simulink model "TermProject_sim"  (R2022a)
settings: Solver=VariableStepAuto  StartTime=0.0  StopTime=3  RelTol=1e-3
values from neighbouring files (symbols this model uses):
  Beq = Jeq/t    (= 0.00458272318505)    [TermProject.m]
  degtorad = pi/180    (= 0.0174532925199)    [TermProject.m]
  Jeq = J+k*JG+k*J_load    (= 1.72310391758e-05)    [TermProject.m]
  Ka_c = 1/Kp_c    (= 1.20938406605)    [TermProject.m]
  Ka_s = 1/Kp_s    (= 31.5427366344)    [TermProject.m]
  Kd_p = wcp/wcs    (= 0.1)    [TermProject.m]
  Ke = Kt    (= 0.0683)    [TermProject.m]
  Ki_c = wcc*Ra    (= 2211.68122813)    [TermProject.m]
  Ki_s = Beq*wcs/Kt    (= 8.43165416785)    [TermProject.m]
  Kp_c = wcc*La    (= 0.826867186425)    [TermProject.m]
  Kp_p = wcp    (= 12.5663706144)    [TermProject.m]
  Kp_s = Jeq*wcs/Kt    (= 0.0317030196711)    [TermProject.m]
  Kt = 68.3*(10^-3)    (= 0.0683)    [TermProject.m]
  La = 0.000658    [TermProject.m]
  N1 = 1    [TermProject.m]
  N2 = 81    [TermProject.m]
  Ra = 1.76    [TermProject.m]
  radtodeg = 180/pi    (= 57.2957795131)    [TermProject.m]
settings Model: Creator=OS  LastModifiedBy=OS

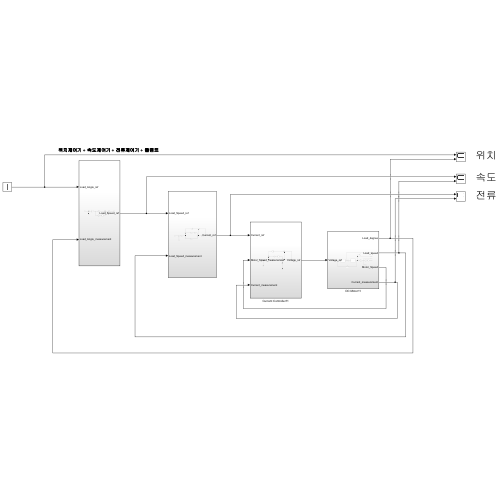
[thumbnail: Simulink's stored preview of the top-level diagram]
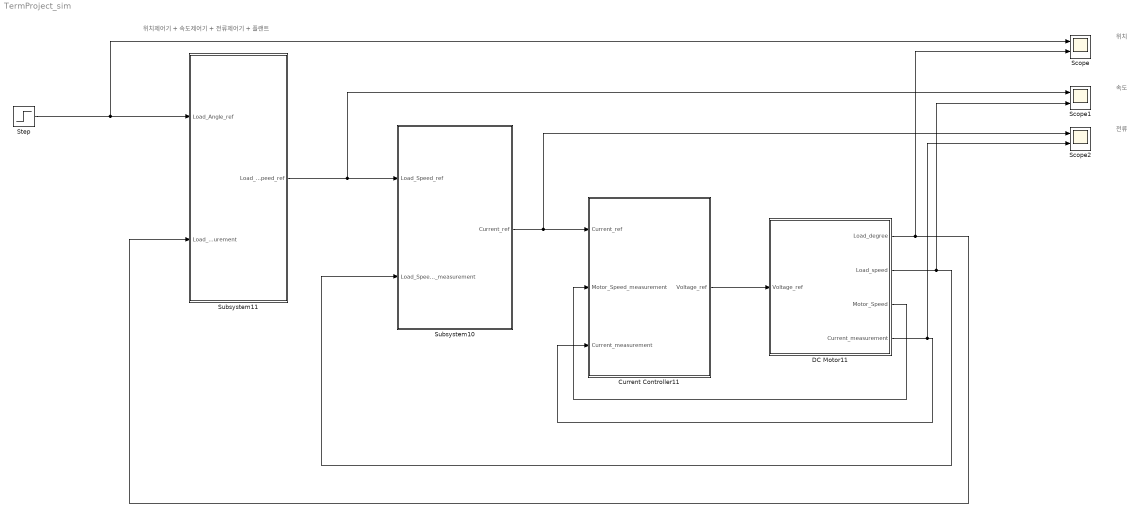
== system TermProject_sim ==
  note: 위치
  note: 위치제어기 + 속도제어기 + 전류제어기 + 플랜트
  note: 속도
  note: 전류
  Current Controller11 : Subsystem
  DC Motor11 : Subsystem
  Scope : Scope  NumInputPorts=2
  Scope1 : Scope  NumInputPorts=2
  Scope2 : Scope  NumInputPorts=2
  Step : Step  After=90  SampleTime=0
  Subsystem10 : Subsystem
  Subsystem11 : Subsystem
  wires:
  DC Motor11/3(Motor_Speed) -> Current Controller11/2(Motor_Speed_measurement)
  Current Controller11/1(Voltage_ref) -> DC Motor11/1(Voltage_ref)
  DC Motor11/4(Current_measurement) -> Scope2/2, Current Controller11/3(Current_measurement)
  DC Motor11/2(Load_speed) -> Scope1/2, Subsystem10/2(Load_Speed_measurement)
  DC Motor11/1(Load_degree) -> Scope/2, Subsystem11/2(Load_Angle_measurement)
  Step/1 -> Subsystem11/1(Load_Angle_ref), Scope/1
  Subsystem10/1(Current_ref) -> Scope2/1, Current Controller11/1(Current_ref)
  Subsystem11/1(Load_Speed_ref) -> Scope1/1, Subsystem10/1(Load_Speed_ref)

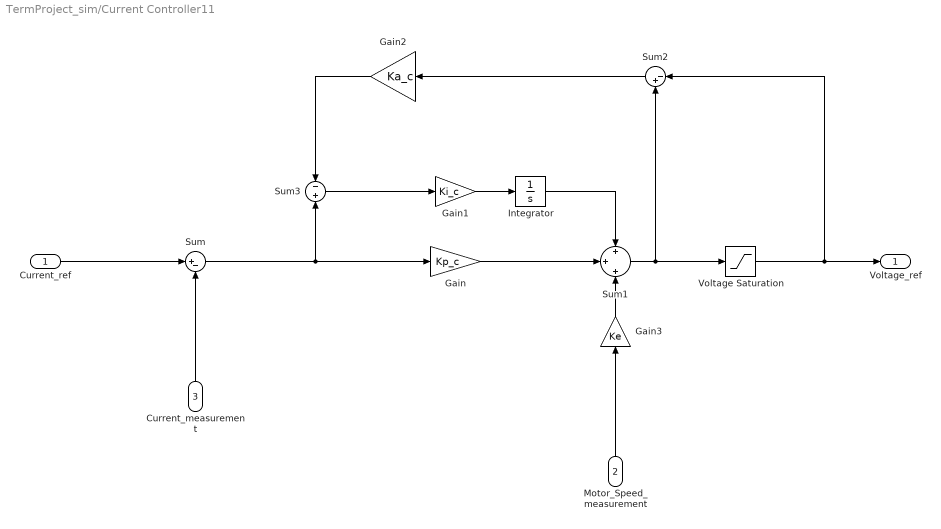
== system TermProject_sim/Current Controller11 ==
  Current_ref : Inport
  Motor_Speed_measurement : Inport  Port=2
  Current_measurement : Inport  Port=3
  Gain : Gain  Gain=Kp_c
  Gain1 : Gain  Gain=Ki_c
  Gain2 : Gain  Gain=Ka_c
  Gain3 : Gain  Gain=Ke
  Integrator : Integrator
  Sum : Sum  Inputs=|+-
  Sum1 : Sum  Inputs=+|+|+
  Sum2 : Sum  Inputs=|-+
  Sum3 : Sum  Inputs=-|+
  Voltage Saturation : Saturate  UpperLimit=48  LowerLimit=-48
  Voltage_ref : Outport
  wires:
  Current_measurement/1 -> Sum/2
  Motor_Speed_measurement/1 -> Gain3/1
  Gain3/1 -> Sum1/3
  Sum2/1 -> Gain2/1
  Gain2/1 -> Sum3/1
  Sum3/1 -> Gain1/1
  Voltage Saturation/1 -> Voltage_ref/1, Sum2/1
  Sum1/1 -> Voltage Saturation/1, Sum2/2
  Gain/1 -> Sum1/2
  Integrator/1 -> Sum1/1
  Gain1/1 -> Integrator/1
  Sum/1 -> Sum3/2, Gain/1
  Current_ref/1 -> Sum/1

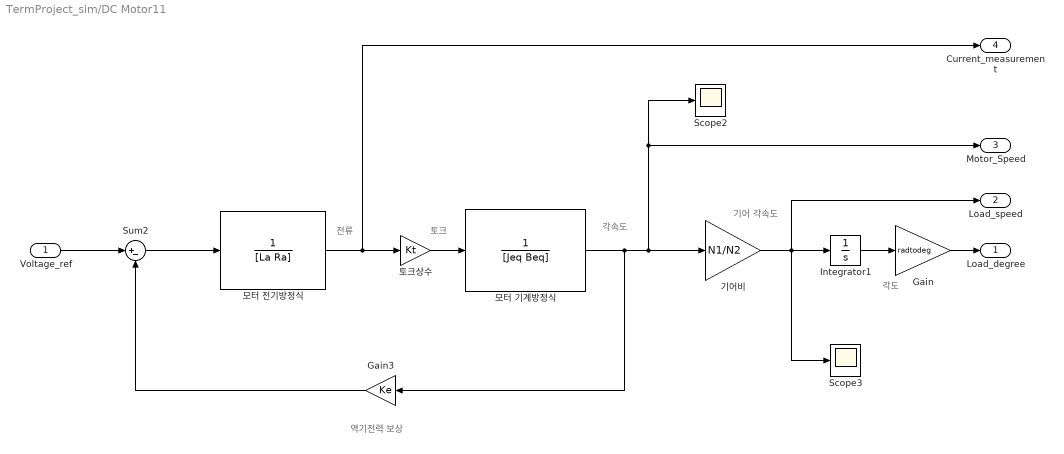
== system TermProject_sim/DC Motor11 ==
  note: 기어 각속도
  note: 각속도
  note: 전류
  note: 토크
  note: 역기전력 보상
  note: 각도
  Voltage_ref : Inport
  Gain : Gain  Gain=radtodeg
  Gain3 : Gain  Gain=Ke
  Integrator1 : Integrator
  Scope2 : Scope
  Scope3 : Scope
  Sum2 : Sum  Inputs=|+-
  기어비 : Gain  Gain=N1/N2
  모터 기계방정식 : TransferFcn  Denominator=[Jeq Beq]
  모터 전기방정식 : TransferFcn  Denominator=[La Ra]
  토크상수 : Gain  Gain=Kt
  Load_degree : Outport
  Load_speed : Outport  Port=2
  Motor_Speed : Outport  Port=3
  Current_measurement : Outport  Port=4
  wires:
  Gain/1 -> Load_degree/1
  Integrator1/1 -> Gain/1
  모터 기계방정식/1 -> Gain3/1, 기어비/1, Motor_Speed/1, Scope2/1
  토크상수/1 -> 모터 기계방정식/1
  Sum2/1 -> 모터 전기방정식/1
  기어비/1 -> Integrator1/1, Scope3/1, Load_speed/1
  Voltage_ref/1 -> Sum2/1
  Gain3/1 -> Sum2/2
  모터 전기방정식/1 -> 토크상수/1, Current_measurement/1

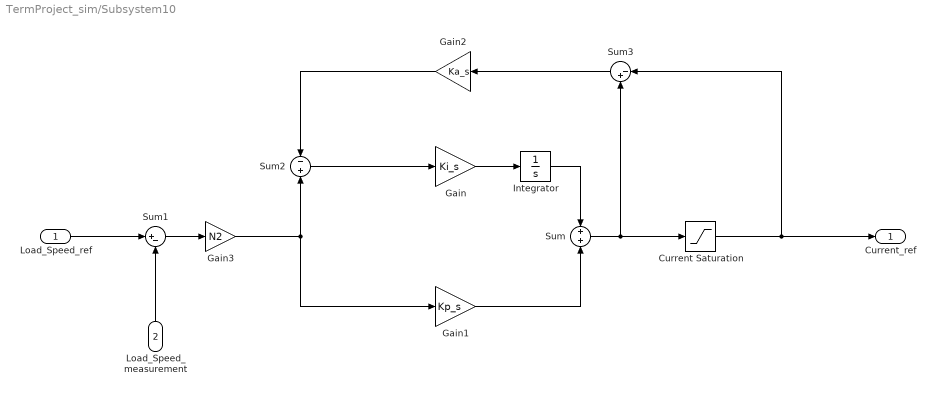
== system TermProject_sim/Subsystem10 ==
  Load_Speed_ref : Inport
  Load_Speed_measurement : Inport  Port=2
  Current Saturation : Saturate  UpperLimit=27.3  LowerLimit=-27.3
  Gain : Gain  Gain=Ki_s
  Gain1 : Gain  Gain=Kp_s
  Gain2 : Gain  Gain=Ka_s
  Gain3 : Gain  Gain=N2
  Integrator : Integrator
  Sum : Sum  Inputs=+|+
  Sum1 : Sum  Inputs=|+-
  Sum2 : Sum  Inputs=-|+
  Sum3 : Sum  Inputs=|-+
  Current_ref : Outport
  wires:
  Integrator/1 -> Sum/1
  Gain/1 -> Integrator/1
  Gain3/1 -> Sum2/2, Gain1/1
  Sum1/1 -> Gain3/1
  Gain1/1 -> Sum/2
  Sum2/1 -> Gain/1
  Load_Speed_measurement/1 -> Sum1/2
  Load_Speed_ref/1 -> Sum1/1
  Gain2/1 -> Sum2/1
  Sum/1 -> Sum3/2, Current Saturation/1
  Sum3/1 -> Gain2/1
  Current Saturation/1 -> Sum3/1, Current_ref/1

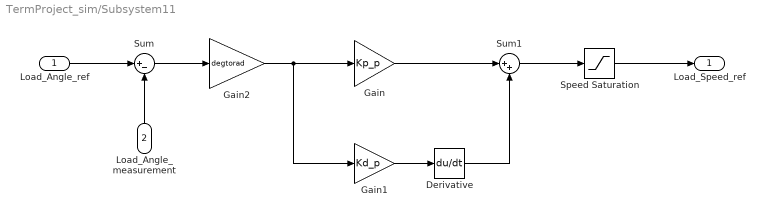
== system TermProject_sim/Subsystem11 ==
  Load_Angle_ref : Inport
  Load_Angle_measurement : Inport  Port=2
  Derivative : Derivative
  Gain : Gain  Gain=Kp_p
  Gain1 : Gain  Gain=Kd_p
  Gain2 : Gain  Gain=degtorad
  Speed Saturation : Saturate  UpperLimit=642.9792964/81  LowerLimit=-642.9792964/81
  Sum : Sum  Inputs=|+-
  Sum1 : Sum  Inputs=|++
  Load_Speed_ref : Outport
  wires:
  Sum1/1 -> Speed Saturation/1
  Speed Saturation/1 -> Load_Speed_ref/1
  Load_Angle_ref/1 -> Sum/1
  Gain/1 -> Sum1/1
  Gain1/1 -> Derivative/1
  Load_Angle_measurement/1 -> Sum/2
  Derivative/1 -> Sum1/2
  Gain2/1 -> Gain1/1, Gain/1
  Sum/1 -> Gain2/1
